simulink model "PLL1_CT"  (R2019b)
settings: Solver=ode23  StartTime=0.0  StopTime=tstop  RelTol=1e-5
values from neighbouring files (symbols this model uses):
  dw = 0.1    [LAB2_script.m]
  Kpd = 1    [LAB2_script.m]
  Kvco = 1    [LAB2_script.m]
  tau = 0.5    [LAB2_script.m]
settings Model: Creator=franc  LastModifiedBy=franc

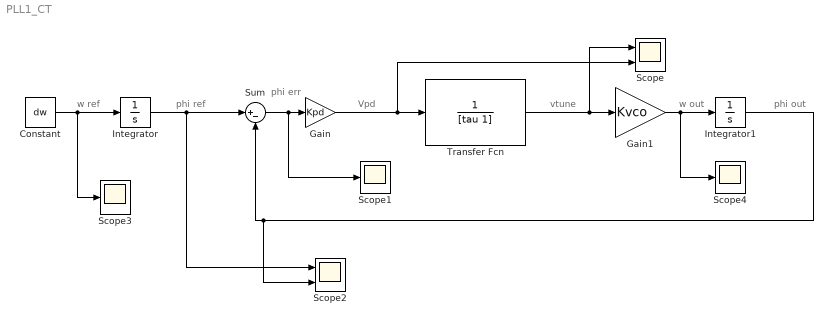
== system PLL1_CT ==
  note: w out
  note: vtune
  note: Vpd
  note: phi err
  note: phi out
  note: phi ref
  note: w ref
  Constant : Constant  Value=dw
  Gain : Gain  Gain=Kpd
  Gain1 : Gain  Gain=Kvco
  Integrator : Integrator
  Integrator1 : Integrator
  Scope : Scope  NumInputPorts=2
  Scope1 : Scope
  Scope2 : Scope  NumInputPorts=2
  Scope3 : Scope
  Scope4 : Scope
  Sum : Sum  Inputs=|+-
  Transfer Fcn : TransferFcn  Denominator=[tau 1]
  wires:
  Constant/1 -> Scope3/1, Integrator/1
  Integrator/1 -> Scope2/1, Sum/1
  Sum/1 -> Scope1/1, Gain/1
  Gain/1 -> Scope/2, Transfer Fcn/1
  Transfer Fcn/1 -> Scope/1, Gain1/1
  Gain1/1 -> Scope4/1, Integrator1/1
  Integrator1/1 -> Scope2/2, Sum/2
